simulink subsystem "modB_sys"  (R2023a)
settings: Solver=VariableStepAuto  StartTime=0.0  StopTime=10.0  RelTol=1e-3
settings Model: Creator=Francesco  LastModifiedBy=Francesco

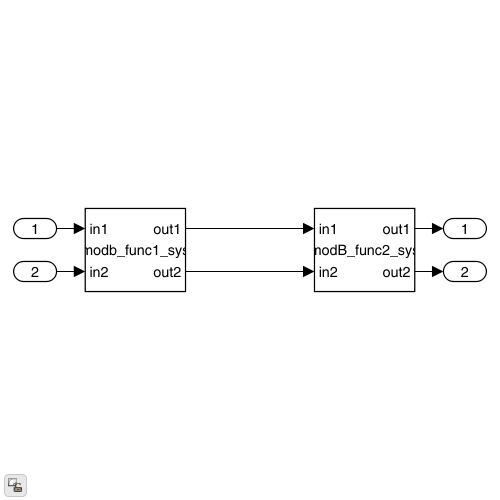
[thumbnail: Simulink's stored preview of the top-level diagram]
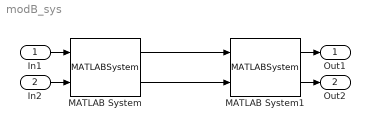
== system modB_sys ==
  In1 : Inport
  In2 : Inport  Port=2
  MATLAB System : MATLABSystem  System=modb_func1_sys  SimulateUsing=Code generation
      mask Type: modb_func1_sys
      mask Display:
      | disp('modb_func1_sys');
      | port_label('input',1,'in1');
      | port_label('input',2,'in2');
      | port_label('output',1,'out1');
      | port_label('output',2,'out2');
  MATLAB System1 : MATLABSystem  System=modB_func2_sys  SimulateUsing=Code generation
      mask Type: modB_func2_sys
      mask Display:
      | disp('modB_func2_sys');
      | port_label('input',1,'in1');
      | port_label('input',2,'in2');
      | port_label('output',1,'out1');
      | port_label('output',2,'out2');
  Out1 : Outport
  Out2 : Outport  Port=2
  wires:
  MATLAB System/1 -> MATLAB System1/1
  MATLAB System/2 -> MATLAB System1/2
  In1/1 -> MATLAB System/1
  MATLAB System1/1 -> Out1/1
  MATLAB System1/2 -> Out2/1
  In2/1 -> MATLAB System/2
